simulink model "C01A_DC_MotorEquation"  (R2025b)
settings: Solver=VariableStepAuto  StartTime=0.0  StopTime=0.2  RelTol=1e-3
values from neighbouring files (symbols this model uses):
  b = (Km*0.3)/((1750*(2*pi))/60)    (= 0.000180072449898)    [C01A_Parameters.m]
  J = 0.352e-4    (= 3.52e-05)    [C01A_Parameters.m]
  Km = 0.11    [C01A_Parameters.m]
  L = 4.1e-3    (= 0.0041)    [C01A_Parameters.m]
  R = 3.2    [C01A_Parameters.m]
  RadToRpm = 60/(2*pi)    (= 9.54929658551)    [C01A_Parameters.m]
settings Model: Creator=Davide  LastModifiedBy=Utente
settings DataIOCC: ReturnWorkspaceOutputs=off
settings OptimizationCC: ReuseModelBlockBuffer=off
settings RTWCC: GPUComputeCapability=3.5

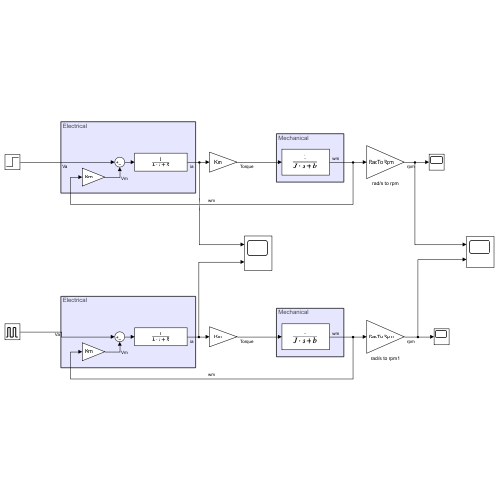
[thumbnail: Simulink's stored preview of the top-level diagram]
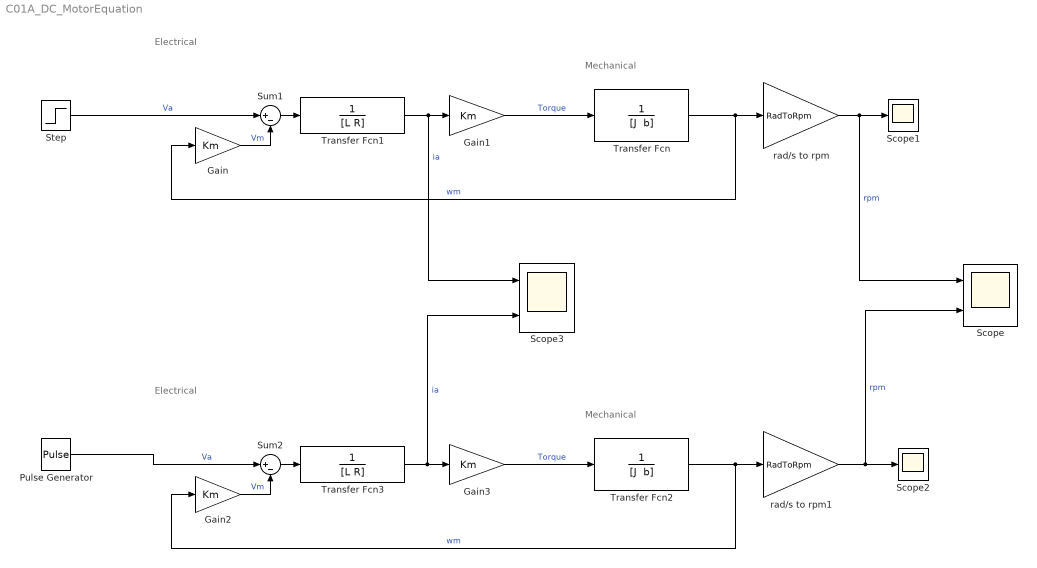
== system C01A_DC_MotorEquation ==
  note: Electrical
  note: Mechanical
  note: Electrical
  note: Mechanical
  Gain{,1..3} (4 alike) : Gain  Gain=Km
  Pulse Generator : DiscretePulseGenerator  PulseType=Time based  Amplitude=24  Period=0.0001  PulseWidth=50
  Scope : Scope  NumInputPorts=2
      settings: ActiveDisplayYMinimum=-124.29833  ActiveDisplayYMaximum=1118.68501
  Scope1 : Scope
      settings: ActiveDisplayYMinimum=-260.43452  ActiveDisplayYMaximum=2343.91067
  Scope2 : Scope
      settings: DataLoggingVariableName=ScopeData2
  Scope3 : Scope  NumInputPorts=2
      settings: ActiveDisplayYMinimum=-0.38599  ActiveDisplayYMaximum=3.4739  DataLoggingVariableName=ScopeData3
  Step : Step  Time=0  After=12  SampleTime=0
  Sum1 : Sum  Inputs=|+-
  Sum2 : Sum  Inputs=|+-
  Transfer Fcn : TransferFcn  Denominator="[J  b]"
  Transfer Fcn1 : TransferFcn  Denominator=[L R]
  Transfer Fcn2 : TransferFcn  Denominator="[J  b]"
  Transfer Fcn3 : TransferFcn  Denominator=[L R]
  rad/s to rpm : Gain  Gain=RadToRpm  SaturateOnIntegerOverflow=on  OutDataTypeStr=Inherit: Same as input  ParamDataTypeStr=Inherit: Same as input
  rad/s to rpm1 : Gain  Gain=RadToRpm  SaturateOnIntegerOverflow=on  OutDataTypeStr=Inherit: Same as input  ParamDataTypeStr=Inherit: Same as input
  wires:
  Gain3/1 -> Transfer Fcn2/1  "Torque"
  rad/s to rpm/1 -> Scope/1, Scope1/1  "rpm"
  Transfer Fcn3/1 -> Scope3/2, Gain3/1  "ia"
  Pulse Generator/1 -> Sum2/1  "Va"
  rad/s to rpm1/1 -> Scope/2, Scope2/1  "rpm"
  Gain/1 -> Sum1/2  "Vm"
  Transfer Fcn1/1 -> Scope3/1, Gain1/1  "ia"
  Transfer Fcn/1 -> rad/s to rpm/1, Gain/1  "wm"
  Sum2/1 -> Transfer Fcn3/1
  Sum1/1 -> Transfer Fcn1/1
  Gain1/1 -> Transfer Fcn/1  "Torque"
  Transfer Fcn2/1 -> rad/s to rpm1/1, Gain2/1  "wm"
  Gain2/1 -> Sum2/2  "Vm"
  Step/1 -> Sum1/1  "Va"
